simulink model "PSO"  (R2020a)
settings: Solver=ode23s  StartTime=0.0  StopTime=2  MaxStep=1e-4  RelTol=1e-3
libraries: powerlib x16, re_lib x5, powerlib_meascontrol x1
settings Model: Creator=Mahesh Krishna  LastModifiedBy=vankurua
settings DataIOCC: ReturnWorkspaceOutputs=off
settings OptimizationCC: LifeSpan=inf
settings DebuggingCC: ArithmeticOperatorsInVariantConditions=warning
settings SFSimCC: SimUseLocalCustomCode=off  CustomCodeUndefinedFunction=UseInterfaceOnly
settings RTWCC: RTWUseLocalCustomCode=off
settings CodeAppCC: StateflowObjectComments=on
settings SimscapeCC: SimscapeNormalizeSystem=off

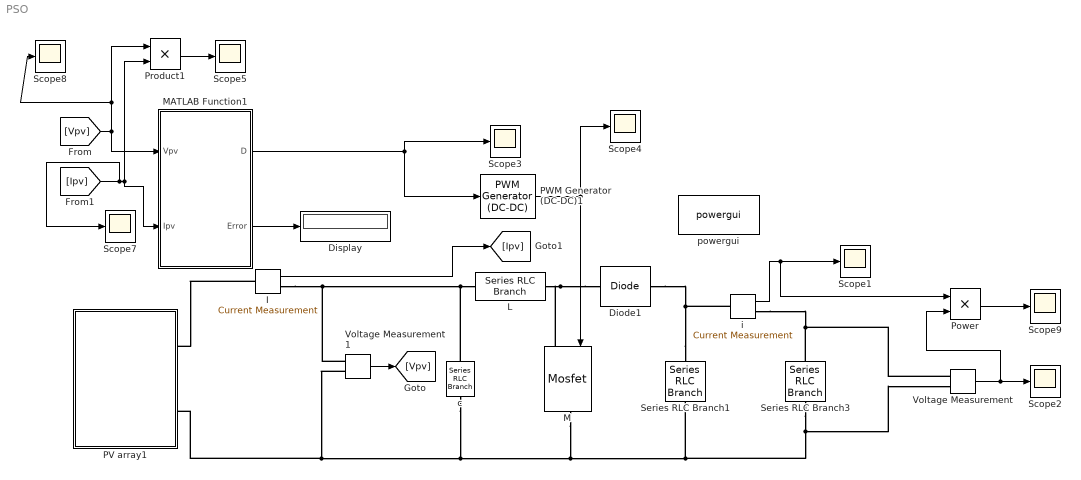
== system PSO ==
  Diode1 : powerlib/Power Electronics/Diode  Ron=1e-3  Lon=0  Vf=0  IC=0  UseSnubber=off  Rs=inf  Cs=inf  Measurements=off
  Display : Display
  I : powerlib/Measurements/Current Measurement  PhasorSimulation=off  OutputType=Magnitude  PSBequivalent=0
  L : powerlib/Elements/Series RLC Branch  LConnTagsString=__new0  RConnTagsString=__new0  BranchType=L  Resistance=1e-3  Inductance=5e-3  SetiL0=off  InitialCurrent=0  Capacitance=1e-6  Setx0=off  InitialVoltage=0  Measurements=None
  M : powerlib/Power Electronics/Mosfet  Ron=1e-3  Lon=0  Rd=1e-3  Vfd=0  IC=0  Rs=inf  Cs=inf  Measurements=off
  MATLAB Function1 : MATLAB Function  TreatAsAtomicUnit=on
  PV array1 : Subsystem
  PWM Generator (DC-DC)1 : powerlib_meascontrol/Pulse & Signal Generators/PWM Generator (DC-DC)  Fsw=20000  Ts=0
  Power : Product
  Product1 : Product
  Scope{1..5,7..9} (8 alike) : Scope
  Series RLC Branch1 : powerlib/Elements/Series RLC Branch  LConnTagsString=__new0  RConnTagsString=__new0  BranchType=C  Resistance=1e-4  Inductance=200e-6  SetiL0=off  InitialCurrent=0  Capacitance=22e-6  Setx0=off  InitialVoltage=40  Measurements=None
  Series RLC Branch3 : powerlib/Elements/Series RLC Branch  LConnTagsString=__new0  RConnTagsString=__new0  BranchType=R  Resistance=100  Inductance=200e-6  SetiL0=off  InitialCurrent=0  Capacitance=1000e-6  Setx0=off  InitialVoltage=40  Measurements=None
  Voltage Measurement : powerlib/Measurements/Voltage Measurement  PhasorSimulation=off  OutputType=Magnitude  PSBequivalent=0
  Voltage Measurement1 : powerlib/Measurements/Voltage Measurement  PhasorSimulation=off  OutputType=Magnitude  PSBequivalent=0
  c : powerlib/Elements/Series RLC Branch  LConnTagsString=__new0  RConnTagsString=__new0  BranchType=C  Resistance=1e-3  Inductance=250e-6  SetiL0=off  InitialCurrent=0  Capacitance=2.2e-6  Setx0=off  InitialVoltage=0  Measurements=None
  i : powerlib/Measurements/Current Measurement  PhasorSimulation=off  OutputType=Magnitude  PSBequivalent=0
  powergui : powerlib/powergui  Priority=1  SimulationMode=Continuous  SampleTime=50e-6  frequency=60  Iterations=50  frequencyindice=0  Pbase=100e6  ErrMax=1e-4  UnitsV=kV  UnitsW=MW  buscounter=0  FunctionMessages=off  echomessages=off  EnableUseOfTLC=off  CurrentSourceSwitches=off  DisableSnubberDevices=off  DisableRonSwitches=off  DisableVfSwitches=off  DisplayEquations=off  AutomaticDiscreteSolvers=off  SolverType=Tustin/Backward Euler (TBE)  Interpol=off  ExternalGateDelay=off  methode=off  Ts=100  x0status=blocks  SPID=on  SwTol=0  HookPort=off  NonlinearTolerance=1e-4  nMaxIteration=100  ContinueOnMaxIteration=off  RestoreLinks=warning  ResistiveCurrentMeasurement=off  Frange=[0:2:500]  Ylog=off  Xlog=on  ShowGrid=off  save=off  variable=ZData  structure=0  ZoomFFT=off  StartTime=0.0  cycles=1  DisplayStyle=1  fundamental=60  FreqAxis=off  MaxFrequency=1000  frequencyindicesteady=1  RmsSteady=1  display=off
  wires:
  I/1 -> [Ipv]
  [Ipv] -> Scope7/1, MATLAB Function1/2(Ipv), Product1/2
  Voltage Measurement/1 -> Power/2, Scope2/1
  PWM Generator (DC-DC)1/1 -> Scope4/1, M/1
  i/1 -> Power/1, Scope1/1
  Voltage Measurement1/1 -> [Vpv]
  [Vpv] -> MATLAB Function1/1(Vpv), Scope8/1, Product1/1
  Product1/1 -> Scope5/1
  Power/1 -> Scope9/1
  MATLAB Function1/1(D) -> Scope3/1, PWM Generator (DC-DC)1/1
  MATLAB Function1/2(Error) -> Display/1
  connections:
  i/RConn1 -- Series RLC Branch3/LConn1 -- Voltage Measurement/LConn1
  Series RLC Branch1/RConn1 -- Series RLC Branch3/RConn1 -- Voltage Measurement/LConn2 -- Voltage Measurement1/LConn2 -- PV array1/RConn2 -- c/RConn1 -- M/RConn1
  Series RLC Branch1/LConn1 -- Diode1/RConn1 -- i/LConn1
  I/LConn1 -- PV array1/RConn1
  Diode1/LConn1 -- M/LConn1 -- L/RConn1
  I/RConn1 -- Voltage Measurement1/LConn1 -- c/LConn1 -- L/LConn1

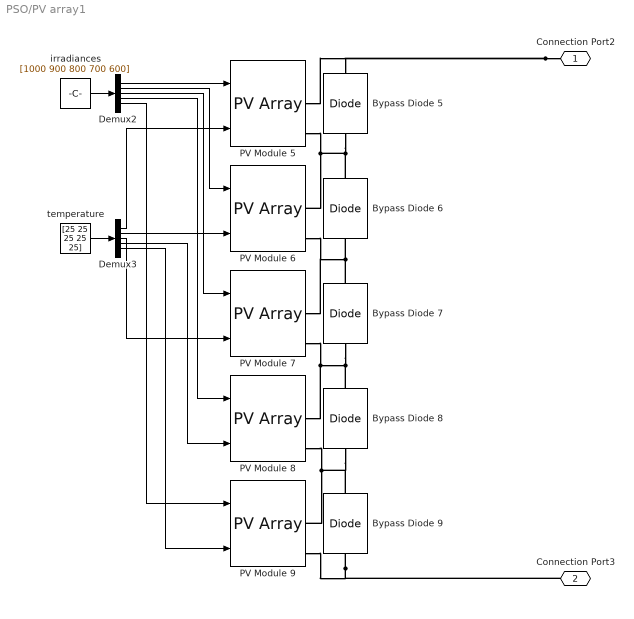
== system PSO/PV array1 ==
  Bypass Diode {5..9} (5 alike) : powerlib/Power Electronics/Diode  Ron=0.001  Lon=0  Vf=0.8  IC=0  UseSnubber=off  Rs=500  Cs=250e-9  Measurements=off
  Demux2 : Demux  Outputs=5
  Demux3 : Demux  Outputs=5
  PV Module 5 : re_lib/Solar/PV Array  Npar=1  Nser=1  PlotType=array @ 25 deg.C & specified irradiances  S_vec="[ 1000  500  100 ]"  Temp_C_vec="[ 45 25  ]"  ModuleName=1Soltech 1STH-215-P  PlotWhenSelected=off  Pm=213.15  Ncell=60  Voc=36.3  Isc=7.84  Vm=29  Im=7.35  beta_Voc_pc=-0.36099  alpha_Isc_pc=0.102  beta_Voc=-0.13104  alpha_Isc=0.007997  IL=7.8649  I0=2.9259e-10  nI=0.98117  Rsh=313.3991  Rs=0.39383  RobustModel=off  RobustCellTemperature=25  BAL=off  Tc=1e-6  Tfilter=5e-5
  PV Module {6..9} (4 alike) : re_lib/Solar/PV Array  Npar=1  Nser=1  PlotType=array @ 1000 W/m2 & specified temperatures  S_vec="[ 1000  500  100 ]"  Temp_C_vec="[ 45 25  ]"  ModuleName=1Soltech 1STH-215-P  PlotWhenSelected=off  Pm=213.15  Ncell=60  Voc=36.3  Isc=7.84  Vm=29  Im=7.35  beta_Voc_pc=-0.36099  alpha_Isc_pc=0.102  beta_Voc=-0.13104  alpha_Isc=0.007997  IL=7.8649  I0=2.9259e-10  nI=0.98117  Rsh=313.3991  Rs=0.39383  RobustModel=off  RobustCellTemperature=25  BAL=off  Tc=1e-6  Tfilter=5e-5
  irradiances : Constant  Value=[1000 900 800 700 600]
  temperature : Constant  Value=[25 25 25 25 25]
  Connection Port2 : PMIOPort  Side=Right
  Connection Port3 : PMIOPort  Port=2  Side=Right
  wires:
  Demux2/1 -> PV Module 5/1
  Demux3/4 -> PV Module 8/2
  Demux3/1 -> PV Module 5/2
  Demux3/3 -> PV Module 7/2
  Demux2/5 -> PV Module 9/1
  Demux2/4 -> PV Module 8/1
  Demux2/3 -> PV Module 7/1
  Demux3/5 -> PV Module 9/2
  irradiances/1 -> Demux2/1
  Demux2/2 -> PV Module 6/1
  temperature/1 -> Demux3/1
  Demux3/2 -> PV Module 6/2
  connections:
  Bypass Diode 6/RConn1 -- Bypass Diode 5/LConn1 -- PV Module 5/RConn2 -- PV Module 6/RConn1
  Connection Port2/RConn1 -- PV Module 5/RConn1 -- Bypass Diode 5/RConn1
  Bypass Diode 9/LConn1 -- Connection Port3/RConn1 -- PV Module 9/RConn2
  Bypass Diode 7/RConn1 -- Bypass Diode 6/LConn1 -- PV Module 7/RConn1 -- PV Module 6/RConn2
  PV Module 8/RConn2 -- PV Module 9/RConn1 -- Bypass Diode 8/LConn1 -- Bypass Diode 9/RConn1
  PV Module 7/RConn2 -- PV Module 8/RConn1 -- Bypass Diode 7/LConn1 -- Bypass Diode 8/RConn1

== matlab function PSO/MATLAB Function1 ==
  settings: updateMethod=DISCRETE  sampleTime=1e-4
  data: Vpv input; D output; Ipv input; Error output
function [D,Error] = PSO(Vpv,Ipv)
    N = 3; %粒子个数
    T = 30; %最大迭代次数
    Xmin = 0; %粒子下限位置
    Xmax = 0.95; %粒子上限位置
    Wmax = 0.8; %惯性权重最大值
    Wmin = 0.4; %惯性权重最小值
    c1 = 1.2; %学习因子 自身对自身的
    c2 = 1.2;  %学习因子 粒子自身对全局最优解的
    
    Vmax = 0.6*((Xmax-Xmin)/2); %速度最大值
    Vmin = -1*Vmax;
    
    %定义种群
    persistent x; %x是群 x(i)是粒子的位置 aka 占空比
    persistent v; %v是群的速度信息 v(i)表示该粒子的速度
    persistent t; %当前的迭代次数
    
    %定义储存适应度的数组
    persistent pbest; %储存的是粒子本身历史上最佳的适应度 aka 功率
    persistent pbposition; %储存的是粒子本身历史最优解的位置 aka 占空比
    
    persistent p; %储存当前种群的适应度 aka 功率
    persistent g; %储存全局最优解位置 aka 占空比
    persistent gbest; %储存全局最优解 aka 功率
    
    persistent counter; %计数的
    persistent u; %当前粒子下标
    persistent dcurrent; %当前或者上一次的占空比
    
    persistent ERROR; %判断有没有ERROR
    
    
    %初始化变量，如果是第一次执行
    if(isempty(x))
        x = rand(N,1)*(Xmax-Xmin)+Xmin;
    end
    if(isempty(v))
        v = rand(N,1)*(Vmax-Vmin)+Vmin;
    end
    if(isempty(t))
        t = 0;
    end
    if(isempty(pbest))
        pbest = zeros(N,1);
    end
    if(isempty(pbest))
        pbest = zeros(N,1);
    end
    if(isempty(pbposition))
        pbposition = zeros(N,1);
    end
    if(isempty(g))
        g = 0;
    end
    if(isempty(p))
        p = zeros(N,1);
    end
    if(isempty(gbest))
        gbest = 0;
    end
    if(isempty(counter))
        counter = 0;
    end
    if(isempty(u))
        u = 0;
    end
    if(isempty(dcurrent))
        dcurrent = 0.5;
    end
    if(isempty(ERROR))
        ERROR = 0;
    end
    %--
    
    Error = ERROR;
    
    %需要150次循环 然后占空比会达到稳定，就是Ipv和Vpv才能稳定
    if(counter>=1 && counter<=150)
        D=dcurrent;
        counter=counter+1;
        return;
    end
    counter = 0;
    
    %实际上是要跑每一个粒子的
    if(u>=1 && u<=N)
       p(u) = Vpv*Ipv; %给u赋值
    end
    
    u=u+1;
    
    
    if(u>=1 && u<=N)
        D=x(u);
        dcurrent=D;
        counter=1;
        return;
    end
    
    
   
    if(u == (N+1)) %需要对粒子群进行计算整理,并且重置种群
        for i=1:N
            if(p(i)>pbest(i)) %如果比pbest(i)，即粒子的历史最优解还要大
                pbest(i) = p(i); %更新粒子历史最优解
                pbposition(i) = x(i); %更新粒子历史最优解位置 aka 占空比
            end
            if(pbest(i)>gbest) %如果大于全局历史最优解
                gbest = pbest(i); %更新全局最优解
                g=x(i); %更新全局最优解位置
            end
            %x(i)是粒子当前的位置 pbposition是粒子目前最优位置
           %还是得考虑动态的惯性权重，不然在逼近最优解的时候波动太大了
           %计算惯性权重
           if(t>=30)
               w=0;
           else
               w = Wmax-(Wmax-Wmin)*t/T;
           end
            
            v(i) = w*v(i)+c1*rand*(pbposition(i)-x(i))+c2*(g-x(i));
            x(i) = x(i)+v(i);
            if(v(i)>Vmax | v(i)<Vmin)
                v(i) = rand * (Vmax-Vmin)+Vmin;
            end
            if(x(i)>Xmax | x(i)<Xmin)
                x(i) = rand * (Xmax-Xmin)+Xmin;
            end
        end
        u=1; %重置u
        D = x(u);
        dcurrent = D;
        counter = 1;
        t=t+1;
        return;
    else
        ERROR=1;
        Error = ERROR;
        D=0.1; 
    end
    
end
